simulink model "MPC"  (R2018a)
settings: Solver=VariableStepAuto  StartTime=0.0  StopTime=15  RelTol=1e-3
values from neighbouring files (symbols this model uses):
  A = [0 1 val.vx 0;0 -2*(val.cf+val.cr)/val.m/val.vx 0 -val.vx-(2*(val.cf*val.lf-val.cr*val.lr)/val.m/val.vx);0 0 0 1;0 -(2*(val.cf*val.lf-val.cr*val.lr))/val.I/val.vx 0 -(2*(val.cf*val.lf^2+val.cr*val.lr^2))/val.I/val.vx]    [ExplicitMPC_code.m]    (also in MPC_code.m = [-2*(val.cf+val.cr)/val.m/val.vx 0 -val.vx-(2*(val.cf*val.lf)
  B = [0 2*val.cf/val.m 0 2*val.lf*val.cf/val.I].'    [ExplicitMPC_code.m]    (also in MPC_code.m = [2*val.cf/val.m 0 2*val.lf*val.cf/val.I 0].')
  C = [1 0 0 0;0 0 1 0]    [ExplicitMPC_code.m]    (also in MPC_code.m = [0 0 0 1; 0 1 0 0])
  D = [0;0]    [ExplicitMPC_code.m]    (also in MPC_code.m)
libraries: mpclib x1
settings Model: Creator=sa2saiye  LastModifiedBy=sa2saiye

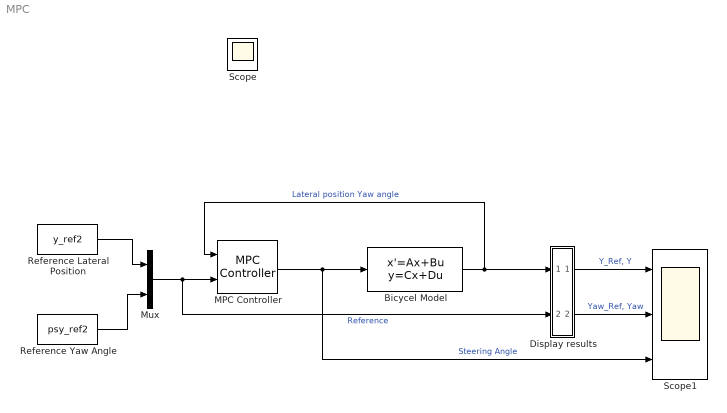
== system MPC ==
  Bicycel Model : StateSpace  A=A  B=B  C=C  D=D  InitialCondition=0
  Display results : Subsystem
  MPC Controller : mpclib/MPC Controller  SCDEnableBlockLinearizationSpecification=on  mpcobj=mpc1  is_multiple=0  enable_value=0  return_u0=off  updateMPCinCallerWorkspace=on  ref_from_ws=off  ref_signal_name=[]  ref_preview=off  md_from_ws=off  md_signal_name=[]  md_preview=off  from_project=off  project_file=MPCtask.mat  md_inport=off  mv_inport=off  cost_outport=off  return_sequence=off  return_qpstatus=off  return_state=off  state_inport=off  lims_inport=off  cc_inport=off  ywt_inport=off  is_designfromscratch=0  uwt_inport=off  duwt_inport=off  rhoeps_inport=off  uref_inport=off  n_ts=0.1  n_p=3  n_mv=1  n_md=0  n_ud=0  n_mo=2  n_uo=0  BlockDataType=double  SampleTimeInherited=off  switch_inport=off
  Mux : Mux  Inputs=2
  Reference Lateral Position : FromWorkspace  VariableName=y_ref2  SampleTime=0.1
  Reference Yaw Angle : FromWorkspace  VariableName=psy_ref2  SampleTime=0.1
  Scope1 : Scope  NumInputPorts=3
  Scope : Scope
  wires:
  MPC Controller/1 -> Scope1/3, Bicycel Model/1  "Steering Angle"
  Reference Lateral Position/1 -> Mux/1
  Bicycel Model/1 -> MPC Controller/1, Display results/1(Outputs)  "Lateral position Yaw angle"
  Display results/2(Out1) -> Scope1/2  "Yaw_Ref, Yaw"
  Reference Yaw Angle/1 -> Mux/2
  Mux/1 -> MPC Controller/2, Display results/2(References)  "Reference"
  Display results/1(Out2) -> Scope1/1  "Y_Ref, Y"

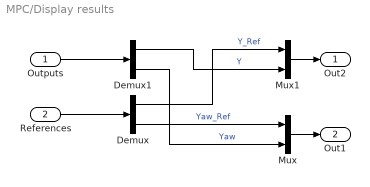
== system MPC/Display results ==
  Outputs : Inport
  References : Inport  Port=2
  Demux : Demux  Outputs=2
  Demux1 : Demux  Outputs=2
  Mux : Mux  Inputs=2
  Mux1 : Mux  Inputs=2
  Out2 : Outport
  Out1 : Outport  Port=2
  wires:
  Demux/2 -> Mux/1  "Yaw_Ref"
  Mux/1 -> Out1/1
  Demux1/1 -> Mux1/2  "Y"
  Demux/1 -> Mux1/1  "Y_Ref"
  Mux1/1 -> Out2/1
  Outputs/1 -> Demux1/1
  References/1 -> Demux/1
  Demux1/2 -> Mux/2  "Yaw"
